simulink model "SF103A_MotorReferenceModel_v001B_MappedToEA4"  (R2013b)
settings: Solver=FixedStepDiscrete  StartTime=0.0  StopTime=10.0  RelTol=1e-3
InitFcn:
  | SF103A_MotorReferenceModel_v001X_Parameters;
undefined symbols (not defined in the file or in its folder): D_DTSCLMAX_ULS, D_DTSCLMIN_ULS, D_VECUMAX_VOLTS, D_VECUMIN_VOLTS, MtrCtrl_d_Ts_slow_s, MtrCtrl_e_KeNom_VpRadpS, MtrCtrl_e_RmNom_Ohm, MtrCtrl_k_deadtimeVScale_Uls, MtrCtrl_k_FeedbackControlDisable_Cnt, MtrCtrl_k_IdBoostGain_Uls, MtrCtrl_k_IdBoostVRThreshScl_Uls, MtrCtrl_k_IdqRefIminTol_Uls, MtrCtrl_k_IdqRefTrqTol_Uls, MtrCtrl_k_LdNom_Henry, MtrCtrl_k_LqNom_Henry, MtrCtrl_k_MtrCurrDaxMaxValScl_Per, MtrCtrl_k_MtrVoltDervFiltTimeConst_Sec, MtrCtrl_k_NoofPoles_Uls, MtrCtrl_k_VoltModeDynCompEnable_Cnt, MtrCtrl_t_IdBoostTrqCharSclY_Uls, MtrCtrl_t_IdBoostTrqCmdX_MtrNm, MtrCtrl_t_IdqRefDeltaPoints_Rad, MtrCtrl_t_Q13VltgSchedXTbl_MtrRadpS, MtrCtrl_t_Q13VltgSchedYTbl_Volt, MtrCtrl_t_Q24VltgSchedXTbl_MtrRadpS, MtrCtrl_t_Q24VltgSchedYTbl_Volt
undefined symbols (not defined in the file): MtrCtrl_k_MtrVelFiltFFKn_Hz
libraries: simulink x6
(part 2 of 2)

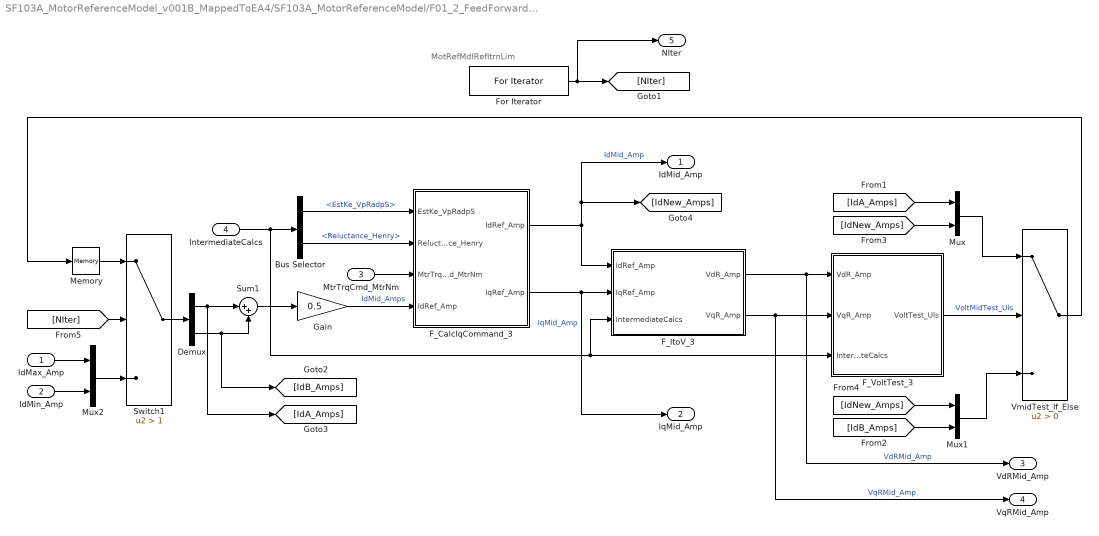
== system SF103A_MotorReferenceModel_v001B_MappedToEA4/SF103A_MotorReferenceModel/F01_2_FeedForward_Reference_Calc/F01_1_6_6_LocateRef/F01_1_6_6_1_ForIteratorSubsystem ==
  note: MotRefMdlRefItrnLim
  IdMax_Amp : Inport
  IdMin_Amp : Inport  Port=2
  MtrTrqCmd_MtrNm : Inport  Port=3
  IntermediateCalcs : Inport  Port=4
  Bus Selector : BusSelector  OutputSignals=EstKe_VpRadpS,Reluctance_Henry
  Demux : Demux  Outputs=2
  F_CalcIqCommand_3 : Subsystem
  F_ItoV_3 : Subsystem
  F_VoltTest_3 : Subsystem
  For Iterator : ForIterator  IterationLimit=MtrCtrl_k_IdqRefLocateRefNIter_Uls
  Gain : Gain  Gain=0.5
  Memory : Memory  InheritSampleTime=on
  Mux : Mux  Inputs=2
  Mux1 : Mux  Inputs=2
  Mux2 : Mux  Inputs=2
  Sum1 : Sum  Inputs=|++
  Switch1 : Switch  Criteria=u2 > Threshold  Threshold=1
  VmidTest_If_Else : Switch  Criteria=u2 > Threshold
  IdMid_Amp : Outport
  IqMid_Amp : Outport  Port=2
  VdRMid_Amp : Outport  Port=3
  VqRMid_Amp : Outport  Port=4
  NIter : Outport  Port=5
  wires:
  Sum1/1 -> Gain/1
  Demux/2 -> [IdB_Amps], Sum1/2
  Demux/1 -> [IdA_Amps], Sum1/1
  Switch1/1 -> Demux/1
  IdMax_Amp/1 -> Mux2/1
  Mux2/1 -> Switch1/3
  IdMin_Amp/1 -> Mux2/2
  [NIter] -> Switch1/2
  Memory/1 -> Switch1/1
  [IdB_Amps] -> Mux1/2
  [IdNew_Amps] -> Mux1/1
  [IdNew_Amps] -> Mux/2
  [IdA_Amps] -> Mux/1
  VmidTest_If_Else/1 -> Memory/1
  Mux1/1 -> VmidTest_If_Else/3
  Mux/1 -> VmidTest_If_Else/1
  For Iterator/1 -> NIter/1, [NIter]
  F_VoltTest_3/1(VoltTest_Uls) -> VmidTest_If_Else/2  "VoltMidTest_Uls"
  F_ItoV_3/2(VqR_Amp) -> F_VoltTest_3/2(VqR_Amp), VqRMid_Amp/1  "VqRMid_Amp"
  F_ItoV_3/1(VdR_Amp) -> F_VoltTest_3/1(VdR_Amp), VdRMid_Amp/1  "VdRMid_Amp"
  F_CalcIqCommand_3/2(IqRef_Amp) -> F_ItoV_3/2(IqRef_Amp), IqMid_Amp/1  "IqMid_Amp"
  F_CalcIqCommand_3/1(IdRef_Amp) -> F_ItoV_3/1(IdRef_Amp), IdMid_Amp/1, [IdNew_Amps]  "IdMid_Amp"
  MtrTrqCmd_MtrNm/1 -> F_CalcIqCommand_3/3(MtrTrqCmd_MtrNm)
  Bus Selector/2 -> F_CalcIqCommand_3/2(Reluctance_Henry)  "<Reluctance_Henry>"
  Bus Selector/1 -> F_CalcIqCommand_3/1(EstKe_VpRadpS)  "<EstKe_VpRadpS>"
  Gain/1 -> F_CalcIqCommand_3/4("IdRef_Amp ")  "IdMid_Amps"
  IntermediateCalcs/1 -> F_ItoV_3/3(IntermediateCalcs), F_VoltTest_3/3(IntermediateCalcs), Bus Selector/1

== system SF103A_MotorReferenceModel_v001B_MappedToEA4/SF103A_MotorReferenceModel/F01_2_FeedForward_Reference_Calc/F01_1_6_6_LocateRef/F_CalcIqCommand_1 ==
  EstKe_VpRadpS : Inport
  Reluctance_Henry : Inport  Port=2
  MtrTrqCmd_MtrNm : Inport  Port=3
  "IdRef_Amp " : Inport  Port=4
  Product : Product  RndMeth=Zero
  Product1 : Product  Inputs=*/  RndMeth=Zero
  Sum : Sum  Inputs=|++
  IdRef_Amp : Outport
  IqRef_Amp : Outport  Port=2
  wires:
  Product1/1 -> IqRef_Amp/1
  MtrTrqCmd_MtrNm/1 -> Product1/1
  Sum/1 -> Product1/2
  Product/1 -> Sum/2
  EstKe_VpRadpS/1 -> Sum/1
  "IdRef_Amp "/1 -> IdRef_Amp/1, Product/2
  Reluctance_Henry/1 -> Product/1

== system SF103A_MotorReferenceModel_v001B_MappedToEA4/SF103A_MotorReferenceModel/F01_2_FeedForward_Reference_Calc/F01_1_6_6_LocateRef/F_ItoV_1  ==
  IdRef_Amp : Inport
  IqRef_Amp : Inport  Port=2
  IntermediateCalcs : Inport  Port=3
  Bus Selector1 : BusSelector  OutputSignals=XqOvrR_Uls,XdOvrR_Uls,EgOvrR_Amp
  Product : Product  RndMeth=Zero
  Product1 : Product  RndMeth=Zero
  Sum : Sum  Inputs=|+-
  Sum1 : Sum  Inputs=+++
  VdR_Amp : Outport
  VqR_Amp : Outport  Port=2
  wires:
  IqRef_Amp/1 -> Product/1, Sum1/1
  IdRef_Amp/1 -> Sum/2, Product1/1
  IntermediateCalcs/1 -> Bus Selector1/1
  Bus Selector1/1 -> Product/2  "<XqOvrR_Uls>"
  Bus Selector1/2 -> Product1/2  "<XdOvrR_Uls>"
  Bus Selector1/3 -> Sum1/3  "<EgOvrR_Amp>"
  Product/1 -> Sum/1
  Sum/1 -> VdR_Amp/1
  Product1/1 -> Sum1/2
  Sum1/1 -> VqR_Amp/1

== system SF103A_MotorReferenceModel_v001B_MappedToEA4/SF103A_MotorReferenceModel/F01_2_FeedForward_Reference_Calc/F01_1_6_6_LocateRef/F_ItoV_2 ==
  IdRef_Amp : Inport
  IqRef_Amp : Inport  Port=2
  IntermediateCalcs : Inport  Port=3
  Bus Selector1 : BusSelector  OutputSignals=XqOvrR_Uls,XdOvrR_Uls,EgOvrR_Amp
  Product : Product  RndMeth=Zero
  Product1 : Product  RndMeth=Zero
  Sum : Sum  Inputs=|+-
  Sum1 : Sum  Inputs=+++
  VdR_Amp : Outport
  VqR_Amp : Outport  Port=2
  wires:
  Sum1/1 -> VqR_Amp/1
  Product1/1 -> Sum1/2
  Sum/1 -> VdR_Amp/1
  Product/1 -> Sum/1
  Bus Selector1/3 -> Sum1/3  "<EgOvrR_Amp>"
  Bus Selector1/2 -> Product1/2  "<XdOvrR_Uls>"
  Bus Selector1/1 -> Product/2  "<XqOvrR_Uls>"
  IntermediateCalcs/1 -> Bus Selector1/1
  IdRef_Amp/1 -> Product1/1, Sum/2
  IqRef_Amp/1 -> Sum1/1, Product/1

== system SF103A_MotorReferenceModel_v001B_MappedToEA4/SF103A_MotorReferenceModel/F01_2_FeedForward_Reference_Calc/F01_1_6_6_LocateRef/F_VoltTest_1 ==
  VdR_Amp : Inport
  VqR_Amp : Inport  Port=2
  IntermediateCalcs : Inport  Port=3
  Bus Selector1 : BusSelector  OutputSignals=VR2_AmpSq
  FALSE : Constant  Value=0
  Math Function : Math  Operator=square  SaturateOnIntegerOverflow=on
  Math Function1 : Math  Operator=square  SaturateOnIntegerOverflow=on
  Sum : Sum  Inputs=|++
  Sum1 : Sum  Inputs=-+|
  Switch : Switch
  TRUE : Constant
  VoltTest_Uls : Outport
  wires:
  IntermediateCalcs/1 -> Bus Selector1/1
  Bus Selector1/1 -> Sum1/1  "<VR2_AmpSq>"
  VdR_Amp/1 -> Math Function/1  "VdR_Amp"
  VqR_Amp/1 -> Math Function1/1  "VqR_Amp"
  Math Function/1 -> Sum/1
  Math Function1/1 -> Sum/2
  Sum/1 -> Sum1/2
  Sum1/1 -> Switch/2
  TRUE/1 -> Switch/1
  FALSE/1 -> Switch/3
  Switch/1 -> VoltTest_Uls/1

== system SF103A_MotorReferenceModel_v001B_MappedToEA4/SF103A_MotorReferenceModel/F01_2_FeedForward_Reference_Calc/F01_1_6_6_LocateRef/F_VoltTest_2 ==
  VdR_Amp : Inport
  VqR_Amp : Inport  Port=2
  IntermediateCalcs : Inport  Port=3
  Bus Selector1 : BusSelector  OutputSignals=VR2_AmpSq
  FALSE : Constant  Value=0
  Math Function : Math  Operator=square  SaturateOnIntegerOverflow=on
  Math Function1 : Math  Operator=square  SaturateOnIntegerOverflow=on
  Sum : Sum  Inputs=|++
  Sum1 : Sum  Inputs=-+|
  Switch : Switch
  TRUE : Constant
  VoltTest_Uls : Outport
  wires:
  Switch/1 -> VoltTest_Uls/1
  FALSE/1 -> Switch/3
  TRUE/1 -> Switch/1
  Sum1/1 -> Switch/2
  Sum/1 -> Sum1/2
  Math Function1/1 -> Sum/2
  Math Function/1 -> Sum/1
  VqR_Amp/1 -> Math Function1/1  "VqR_Amp"
  VdR_Amp/1 -> Math Function/1  "VdR_Amp"
  Bus Selector1/1 -> Sum1/1  "<VR2_AmpSq>"
  IntermediateCalcs/1 -> Bus Selector1/1

== system SF103A_MotorReferenceModel_v001B_MappedToEA4/SF103A_MotorReferenceModel/F01_2_FeedForward_Reference_Calc/F01_1_6_7_DAxisCurrentBoost/F_CalcIqCommand ==
  EstKe_VpRadpS : Inport
  Reluctance_Henry : Inport  Port=2
  MtrTrqCmd_MtrNm : Inport  Port=3
  "IdRef_Amp " : Inport  Port=4
  Product : Product  RndMeth=Zero
  Product1 : Product  Inputs=*/  RndMeth=Zero
  Sum : Sum  Inputs=|++
  IdRef_Amp : Outport
  IqRef_Amp : Outport  Port=2
  wires:
  Product1/1 -> IqRef_Amp/1
  MtrTrqCmd_MtrNm/1 -> Product1/1
  Sum/1 -> Product1/2
  Product/1 -> Sum/2
  EstKe_VpRadpS/1 -> Sum/1
  "IdRef_Amp "/1 -> IdRef_Amp/1, Product/2
  Reluctance_Henry/1 -> Product/1

== system SF103A_MotorReferenceModel_v001B_MappedToEA4/SF103A_MotorReferenceModel/F01_2_FeedForward_Reference_Calc/F01_1_6_7_DAxisCurrentBoost/F_ItoV  ==
  IdRef_Amp : Inport
  IqRef_Amp : Inport  Port=2
  IntermediateCalcs : Inport  Port=3
  Bus Selector1 : BusSelector  OutputSignals=XqOvrR_Uls,XdOvrR_Uls,EgOvrR_Amp
  Product : Product  RndMeth=Zero
  Product1 : Product  RndMeth=Zero
  Sum : Sum  Inputs=|+-
  Sum1 : Sum  Inputs=+++
  VdR_Amp : Outport
  VqR_Amp : Outport  Port=2
  wires:
  IqRef_Amp/1 -> Product/1, Sum1/1
  IdRef_Amp/1 -> Sum/2, Product1/1
  IntermediateCalcs/1 -> Bus Selector1/1
  Bus Selector1/1 -> Product/2  "<XqOvrR_Uls>"
  Bus Selector1/2 -> Product1/2  "<XdOvrR_Uls>"
  Bus Selector1/3 -> Sum1/3  "<EgOvrR_Amp>"
  Product/1 -> Sum/1
  Sum/1 -> VdR_Amp/1
  Product1/1 -> Sum1/2
  Sum1/1 -> VqR_Amp/1

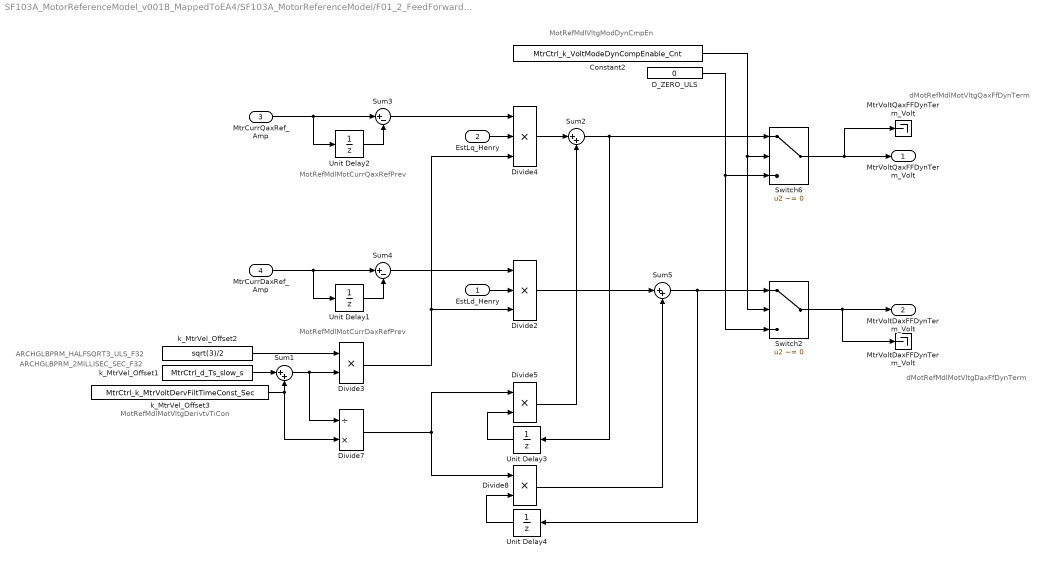
== system SF103A_MotorReferenceModel_v001B_MappedToEA4/SF103A_MotorReferenceModel/F01_2_FeedForward_Reference_Calc/F01_1_6_8_FeedforwardVoltage/F01_1_6_8_1_DynamicTermCalc ==
  note: MotRefMdlMotCurrQaxRefPrev
  note: MotRefMdlVltgModDynCmpEn
  note: MotRefMdlMotVltgDerivtvTiCon
  note: dMotRefMdlMotVltgQaxFfDynTerm
  note: dMotRefMdlMotVltgDaxFfDynTerm
  note: MotRefMdlMotCurrDaxRefPrev
  note: ARCHGLBPRM_HALFSQRT3_ULS_F32
  note: ARCHGLBPRM_2MILLISEC_SEC_F32
  EstLd_Henry : Inport
  EstLq_Henry : Inport  Port=2
  MtrCurrQaxRef_Amp : Inport  Port=3
  MtrCurrDaxRef_Amp : Inport  Port=4
  Constant2 : Constant  Value=MtrCtrl_k_VoltModeDynCompEnable_Cnt
  D_ZERO_ULS : Constant  Value=0
  Divide2 : Product  Inputs=3
  Divide3 : Product
  Divide4 : Product  Inputs=3
  Divide5 : Product
  Divide7 : Product  Inputs=/*
  Divide8 : Product
  "MtrVoltDaxFFDynTerm_Volt " : Terminator
  "MtrVoltQaxFFDynTerm_Volt " : Terminator
  Sum1 : Sum  Inputs=|++
  Sum2 : Sum  Inputs=|++
  Sum3 : Sum  Inputs=|+-
  Sum4 : Sum  Inputs=|+-
  Sum5 : Sum  Inputs=|++
  Switch2 : Switch  Criteria=u2 ~= 0
  Switch6 : Switch  Criteria=u2 ~= 0
  Unit Delay{1..4} (4 alike) : UnitDelay  SampleTime=-1
  k_MtrVel_Offset1 : Constant  Value=MtrCtrl_d_Ts_slow_s  SampleTime=MtrCtrl_d_Ts_slow_s
  k_MtrVel_Offset2 : Constant  Value=sqrt(3)/2  SampleTime=MtrCtrl_d_Ts_slow_s
  k_MtrVel_Offset3 : Constant  Value=MtrCtrl_k_MtrVoltDervFiltTimeConst_Sec  SampleTime=MtrCtrl_d_Ts_slow_s
  MtrVoltQaxFFDynTerm_Volt : Outport
  MtrVoltDaxFFDynTerm_Volt : Outport  Port=2
  wires:
  Sum2/1 -> Unit Delay3/1, Switch6/1
  EstLd_Henry/1 -> Divide2/2
  k_MtrVel_Offset2/1 -> Divide3/1
  k_MtrVel_Offset1/1 -> Sum1/1
  Sum1/1 -> Divide7/1, Divide3/2
  k_MtrVel_Offset3/1 -> Divide7/2, Sum1/2
  EstLq_Henry/1 -> Divide4/2
  Divide3/1 -> Divide4/3, Divide2/3
  Divide4/1 -> Sum2/1
  MtrCurrQaxRef_Amp/1 -> Unit Delay2/1, Sum3/1
  Unit Delay2/1 -> Sum3/2
  Sum3/1 -> Divide4/1
  MtrCurrDaxRef_Amp/1 -> Sum4/1, Unit Delay1/1
  Unit Delay1/1 -> Sum4/2
  Sum4/1 -> Divide2/1
  Divide7/1 -> Divide5/1, Divide8/1
  Divide5/1 -> Sum2/2
  Unit Delay3/1 -> Divide5/2
  Divide2/1 -> Sum5/1
  Unit Delay4/1 -> Divide8/2
  Divide8/1 -> Sum5/2
  Sum5/1 -> Unit Delay4/1, Switch2/1
  Constant2/1 -> Switch2/2, Switch6/2
  D_ZERO_ULS/1 -> Switch6/3, Switch2/3
  Switch6/1 -> "MtrVoltQaxFFDynTerm_Volt "/1, MtrVoltQaxFFDynTerm_Volt/1
  Switch2/1 -> "MtrVoltDaxFFDynTerm_Volt "/1, MtrVoltDaxFFDynTerm_Volt/1

== system SF103A_MotorReferenceModel_v001B_MappedToEA4/SF103A_MotorReferenceModel/F01_2_FeedForward_Reference_Calc/F01_1_6_8_FeedforwardVoltage/F01_1_6_8_2_FeedforwardSelection ==
  note: MotRefMdlFbCtrlDi
  note: dMotRefMdlMotVltgQaxFfDyn
  note: dMotRefMdlMotVltgDaxFfDyn
  MtrVoltDaxFFStatic_Volt : Inport
  MtrVoltQaxFFStatic_Volt : Inport  Port=2
  FailOperActive_Cnt : Inport  Port=3
  MtrVoltQaxFFDynTerm_Volt : Inport  Port=4
  MtrVoltDaxFFDynTerm_Volt : Inport  Port=5
  IntermediateCalcs : Inport  Port=6
  Bus Selector : BusSelector  OutputSignals=EgOvrR_Amp,EstR_Ohm
  D_ZERO_ULS : Constant  Value=0  SampleTime=MtrCtrl_d_Ts_slow_s
  Logical Operator : Logic  Operator=OR  AllPortsSameDT=off  OutDataTypeStr=boolean
  MtrVoltDaxFFDynamic_Volt : Terminator
  "MtrVoltDaxFF_Volt " : Terminator
  MtrVoltQaxFFDynamic_Volt : Terminator
  "MtrVoltQaxFF_Volt " : Terminator
  Product : Product  RndMeth=Zero
  Sum1 : Sum  Inputs=|++
  Sum5 : Sum  Inputs=|++
  Switch1 : Switch  Criteria=u2 ~= 0  SampleTime=MtrCtrl_d_Ts_slow_s
  Switch4 : Switch  Criteria=u2 ~= 0  SampleTime=MtrCtrl_d_Ts_slow_s
  k_MtrVel_Offset9 : Constant  Value=MtrCtrl_k_FeedbackControlDisable_Cnt  SampleTime=MtrCtrl_d_Ts_slow_s
  MtrVoltDaxFF_Volt : Outport
  MtrVoltQaxFF_Volt : Outport  Port=2
  wires:
  Sum5/1 -> Switch1/1, MtrVoltDaxFFDynamic_Volt/1
  Sum1/1 -> MtrVoltQaxFFDynamic_Volt/1, Switch4/1
  Logical Operator/1 -> Switch1/2, Switch4/2
  Switch1/1 -> "MtrVoltDaxFF_Volt "/1, MtrVoltDaxFF_Volt/1
  Switch4/1 -> "MtrVoltQaxFF_Volt "/1, MtrVoltQaxFF_Volt/1
  Product/1 -> Switch4/3
  Bus Selector/2 -> Product/2  "<EstR_Ohm>"
  Bus Selector/1 -> Product/1  "<EgOvrR_Amp>"
  IntermediateCalcs/1 -> Bus Selector/1
  D_ZERO_ULS/1 -> Switch1/3
  k_MtrVel_Offset9/1 -> Logical Operator/1
  FailOperActive_Cnt/1 -> Logical Operator/2
  MtrVoltDaxFFStatic_Volt/1 -> Sum5/1
  MtrVoltDaxFFDynTerm_Volt/1 -> Sum5/2
  MtrVoltQaxFFDynTerm_Volt/1 -> Sum1/2
  MtrVoltQaxFFStatic_Volt/1 -> Sum1/1

== system SF103A_MotorReferenceModel_v001B_MappedToEA4/SF103A_MotorReferenceModel/F01_2_FeedForward_Reference_Calc/F01_1_6_3_LocateTorqueExtremes/F01_1_6_3_3_ChooseDeltaBrackets/F_CalculateTorque ==
  Current : Inport
  IntermediateCalcs : Inport  Port=2
  Bus Selector : BusSelector  OutputSignals=EstKe_VpRadpS,Reluctance_Henry
  Bus Selector1 : BusSelector  OutputSignals=IdRef_Amp,IqRef_Amp
  Product : Product  RndMeth=Zero
  Product1 : Product  RndMeth=Zero
  Sum : Sum  Inputs=++|
  Torque_MtrNm : Outport
  wires:
  Product1/1 -> Torque_MtrNm/1
  Sum/1 -> Product1/1
  Bus Selector1/2 -> Product1/2  "<IqRef_Amp>"
  Bus Selector1/1 -> Product/2  "<IdRef_Amp>"
  Product/1 -> Sum/2
  Current/1 -> Bus Selector1/1
  Bus Selector/2 -> Product/1  "<Reluctance_Henry>"
  Bus Selector/1 -> Sum/1  "<EstKe_VpRadpS>"
  IntermediateCalcs/1 -> Bus Selector/1

== system SF103A_MotorReferenceModel_v001B_MappedToEA4/SF103A_MotorReferenceModel/F01_2_FeedForward_Reference_Calc/F01_1_6_3_LocateTorqueExtremes/F01_1_6_3_3_ChooseDeltaBrackets/F_VSinCosToIdIq ==
  SinDelta : Inport
  CosDelta : Inport  Port=2
  IntermediateCalcs : Inport  Port=3
  Bus Creator : BusCreator  Inputs=2
  Bus Selector2 : BusSelector  OutputSignals=XdOvrR_Uls,VOvrROvrZ_Amp,EgOvrROvrZ_Amp,XqOvrR_Uls,VOvrR_Amp
  Product{,1..3} (4 alike) : Product  RndMeth=Zero
  Sum : Sum  Inputs=|++
  Sum1 : Sum  Inputs=|+-
  Sum2 : Sum  Inputs=|+-
  IdIq_Amp : Outport
  wires:
  Bus Creator/1 -> IdIq_Amp/1
  Sum2/1 -> Bus Creator/2  "IdRef_Amp"
  Product3/1 -> Sum2/2
  Product2/1 -> Sum2/1
  Sum1/1 -> Bus Creator/1, Product2/1  "IqRef_Amp"
  Product1/1 -> Sum1/1
  Sum/1 -> Product1/1
  Product/1 -> Sum/1
  CosDelta/1 -> Sum/2
  SinDelta/1 -> Product3/2, Product/1
  Bus Selector2/5 -> Product3/1  "<VOvrR_Amp>"
  Bus Selector2/4 -> Product2/2  "<XqOvrR_Uls>"
  Bus Selector2/3 -> Sum1/2  "<EgOvrROvrZ_Amp>"
  Bus Selector2/1 -> Product/2  "<XdOvrR_Uls>"
  Bus Selector2/2 -> Product1/2  "<VOvrROvrZ_Amp>"
  IntermediateCalcs/1 -> Bus Selector2/1

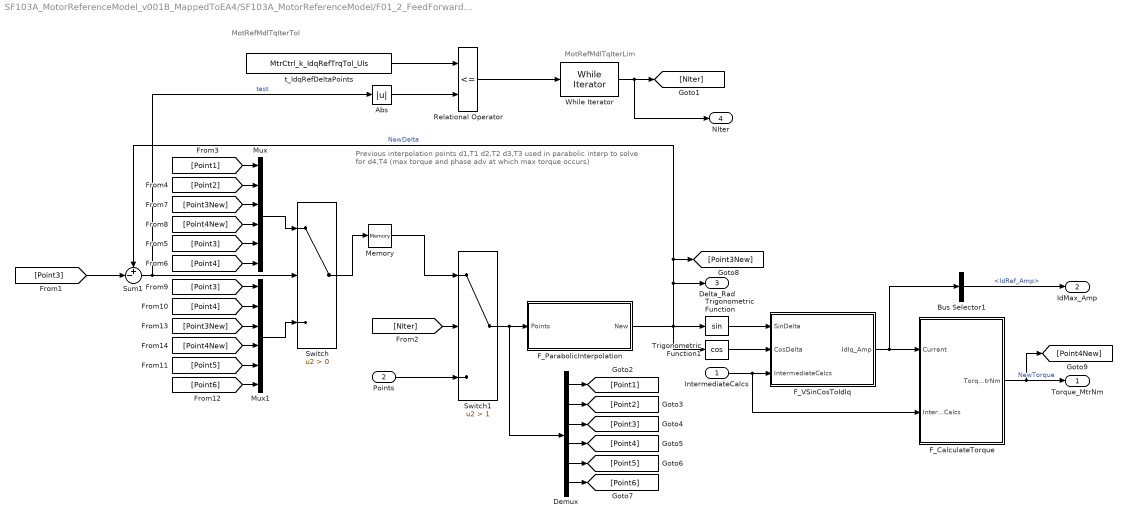
== system SF103A_MotorReferenceModel_v001B_MappedToEA4/SF103A_MotorReferenceModel/F01_2_FeedForward_Reference_Calc/F01_1_6_3_LocateTorqueExtremes/F01_1_6_3_5_InterpolatePeakTorque/F01_1_6_3_5_1_WhileIteratorSubsystem ==
  note: MotRefMdlTqIterLim
  note: Previous interpolation points
      | d1,T1
      | d2,T2
      | d3,T3
      | used in parabolic interp to solve for
      | d4,T4 (max torque and phase adv at which max torque occurs)
  note: MotRefMdlTqIterTol
  IntermediateCalcs : Inport
  Points : Inport  Port=2
  Abs : Abs
  Bus Selector1 : BusSelector  OutputSignals=IdRef_Amp
  Demux : Demux  Outputs=6
  F_CalculateTorque : Subsystem
  F_ParabolicInterpolation : Subsystem
  F_VSinCosToIdIq : Subsystem
  Memory : Memory  InheritSampleTime=on
  Mux : Mux  Inputs=6
  Mux1 : Mux  Inputs=6
  Relational Operator : RelationalOperator  Operator=<=  OutDataTypeStr=boolean
  Sum1 : Sum  Inputs=+-|
  Switch : Switch  Criteria=u2 > Threshold
  Switch1 : Switch  Criteria=u2 > Threshold  Threshold=1
  Trigonometric Function : Trigonometry
  Trigonometric Function1 : Trigonometry  Operator=cos
  While Iterator : WhileIterator  MaxIters=MtrCtrl_k_IdqRefTrqNIter_Uls  WhileBlockType=do-while  ShowIterationPort=on
  t_IdqRefDeltaPoints : Constant  Value=MtrCtrl_k_IdqRefTrqTol_Uls
  Torque_MtrNm : Outport
  IdMax_Amp : Outport  Port=2
  Delta_Rad : Outport  Port=3
  NIter : Outport  Port=4
  wires:
  t_IdqRefDeltaPoints/1 -> Relational Operator/1
  Mux1/1 -> Switch/3
  [Point4New] -> Mux1/4
  [Point3New] -> Mux1/3
  [Point6] -> Mux1/6
  [Point5] -> Mux1/5
  [Point3] -> Mux1/1
  [Point4] -> Mux1/2
  [Point4New] -> Mux/4
  [Point3New] -> Mux/3
  [Point4] -> Mux/6
  [Point3] -> Mux/5
  [Point1] -> Mux/1
  [Point2] -> Mux/2
  [Point3] -> Sum1/2
  Demux/6 -> [Point6]
  Demux/5 -> [Point5]
  Demux/4 -> [Point4]
  Demux/3 -> [Point3]
  Demux/2 -> [Point2]
  Demux/1 -> [Point1]
  Memory/1 -> Switch1/1
  Bus Selector1/1 -> IdMax_Amp/1  "<IdRef_Amp>"
  Points/1 -> Switch1/3
  [NIter] -> Switch1/2
  Switch1/1 -> F_ParabolicInterpolation/1(Points), Demux/1
  While Iterator/1 -> NIter/1, [NIter]
  Switch/1 -> Memory/1
  Mux/1 -> Switch/1
  F_CalculateTorque/1(Torque_MtrNm) -> [Point4New], Torque_MtrNm/1  "NewTorque"
  Abs/1 -> Relational Operator/2
  Sum1/1 -> Abs/1, Switch/2  "test"
  F_VSinCosToIdIq/1(IdIq_Amp) -> Bus Selector1/1, F_CalculateTorque/1(Current)
  IntermediateCalcs/1 -> F_CalculateTorque/2(IntermediateCalcs), F_VSinCosToIdIq/3(IntermediateCalcs)
  Trigonometric Function1/1 -> F_VSinCosToIdIq/2(CosDelta)
  Trigonometric Function/1 -> F_VSinCosToIdIq/1(SinDelta)
  F_ParabolicInterpolation/1(New) -> Trigonometric Function1/1, Sum1/1, [Point3New], Delta_Rad/1, Trigonometric Function/1  "NewDelta"
  Relational Operator/1 -> While Iterator/1

== system SF103A_MotorReferenceModel_v001B_MappedToEA4/SF103A_MotorReferenceModel/F01_2_FeedForward_Reference_Calc/F01_1_6_5_LocateMinIm/F01_1_6_5_1_WhileIteratorSubsystem/F_CalcIqCommand_3 ==
  EstKe_VpRadpS : Inport
  Reluctance_Henry : Inport  Port=2
  MtrTrqCmd_MtrNm : Inport  Port=3
  "IdRef_Amp " : Inport  Port=4
  Product : Product  RndMeth=Zero
  Product1 : Product  Inputs=*/  RndMeth=Zero
  Sum : Sum  Inputs=|++
  IdRef_Amp : Outport
  IqRef_Amp : Outport  Port=2
  wires:
  Reluctance_Henry/1 -> Product/1
  "IdRef_Amp "/1 -> Product/2, IdRef_Amp/1
  EstKe_VpRadpS/1 -> Sum/1
  Product/1 -> Sum/2
  Sum/1 -> Product1/2
  MtrTrqCmd_MtrNm/1 -> Product1/1
  Product1/1 -> IqRef_Amp/1

== system SF103A_MotorReferenceModel_v001B_MappedToEA4/SF103A_MotorReferenceModel/F01_2_FeedForward_Reference_Calc/F01_1_6_5_LocateMinIm/F01_1_6_5_1_WhileIteratorSubsystem/F_ImVSIdq_3 ==
  IdRef_Amp : Inport
  IqRef_Amp : Inport  Port=2
  Math Function : Math  Operator=square  SaturateOnIntegerOverflow=on
  Math Function1 : Math  Operator=square  SaturateOnIntegerOverflow=on
  Sum : Sum  Inputs=|++
  ImRefSq_AmpSq : Outport
  wires:
  IqRef_Amp/1 -> Math Function/1
  IdRef_Amp/1 -> Math Function1/1
  Math Function/1 -> Sum/1
  Math Function1/1 -> Sum/2
  Sum/1 -> ImRefSq_AmpSq/1

== system SF103A_MotorReferenceModel_v001B_MappedToEA4/SF103A_MotorReferenceModel/F01_2_FeedForward_Reference_Calc/F01_1_6_5_LocateMinIm/F01_1_6_5_1_WhileIteratorSubsystem/F_ParabolicInterpolation ==
  note: ARCHGLBPRM_FLOATZEROTHD_ULS_F32
  note: This function checks for
      | divide-by-zero condition
  Points : Inport
  Constant : Constant  Value=eps
  Demux : Demux  Outputs=6
  Gain : Gain  Gain=0.5
  Math Function : Math  Operator=square  SaturateOnIntegerOverflow=on
  Math Function1 : Math  Operator=square  SaturateOnIntegerOverflow=on
  Product{,1..3} (4 alike) : Product  RndMeth=Zero
  Product4 : Product  Inputs=*/  RndMeth=Zero
  Sum{,1..3,5} (5 alike) : Sum  Inputs=|+-
  Sum4 : Sum  Inputs=|++
  Sum6 : Sum  Inputs=|++
  Switch : Switch  Criteria=u2 ~= 0
  New : Outport
  wires:
  Switch/1 -> Product4/2
  Product4/1 -> Gain/1
  Constant/1 -> Switch/3
  Sum5/1 -> Switch/2, Switch/1  "den"
  Points/1 -> Demux/1
  Sum6/1 -> New/1
  Demux/2 -> Sum/1  "Point2:Torque"
  Demux/6 -> Sum1/2  "Point6:Torque"
  Demux/5 -> Sum3/2  "Point5:Delta"
  Demux/4 -> Sum/2, Sum1/1  "Point4:Torque"
  Demux/3 -> Sum3/1, Sum2/2, Sum6/2  "Point3:Delta"
  Demux/1 -> Sum2/1  "Point1:Delta"
  Gain/1 -> Sum6/1
  Product3/1 -> Sum5/2  "den2"
  Product2/1 -> Sum5/1  "den1"
  Sum4/1 -> Product4/1  "num"
  Product1/1 -> Sum4/2  "num2"
  Math Function1/1 -> Product1/2
  Product/1 -> Sum4/1  "num1"
  Math Function/1 -> Product/1
  Sum3/1 -> Product3/2, Math Function1/1  "x2"
  Sum2/1 -> Product2/2, Math Function/1  "x1"
  Sum1/1 -> Product2/1, Product/2  "f2"
  Sum/1 -> Product3/1, Product1/1  "f1"

== system SF103A_MotorReferenceModel_v001B_MappedToEA4/SF103A_MotorReferenceModel/F01_2_FeedForward_Reference_Calc/F01_1_6_6_LocateRef/F01_1_6_6_1_ForIteratorSubsystem/F_CalcIqCommand_3 ==
  EstKe_VpRadpS : Inport
  Reluctance_Henry : Inport  Port=2
  MtrTrqCmd_MtrNm : Inport  Port=3
  "IdRef_Amp " : Inport  Port=4
  Product : Product  RndMeth=Zero
  Product1 : Product  Inputs=*/  RndMeth=Zero
  Sum : Sum  Inputs=|++
  IdRef_Amp : Outport
  IqRef_Amp : Outport  Port=2
  wires:
  Reluctance_Henry/1 -> Product/1
  "IdRef_Amp "/1 -> Product/2, IdRef_Amp/1
  EstKe_VpRadpS/1 -> Sum/1
  Product/1 -> Sum/2
  Sum/1 -> Product1/2
  MtrTrqCmd_MtrNm/1 -> Product1/1
  Product1/1 -> IqRef_Amp/1

== system SF103A_MotorReferenceModel_v001B_MappedToEA4/SF103A_MotorReferenceModel/F01_2_FeedForward_Reference_Calc/F01_1_6_6_LocateRef/F01_1_6_6_1_ForIteratorSubsystem/F_ItoV_3 ==
  IdRef_Amp : Inport
  IqRef_Amp : Inport  Port=2
  IntermediateCalcs : Inport  Port=3
  Bus Selector1 : BusSelector  OutputSignals=XqOvrR_Uls,XdOvrR_Uls,EgOvrR_Amp
  Product : Product  RndMeth=Zero
  Product1 : Product  RndMeth=Zero
  Sum : Sum  Inputs=|+-
  Sum1 : Sum  Inputs=+++
  VdR_Amp : Outport
  VqR_Amp : Outport  Port=2
  wires:
  IqRef_Amp/1 -> Product/1, Sum1/1
  IdRef_Amp/1 -> Sum/2, Product1/1
  IntermediateCalcs/1 -> Bus Selector1/1
  Bus Selector1/1 -> Product/2  "<XqOvrR_Uls>"
  Bus Selector1/2 -> Product1/2  "<XdOvrR_Uls>"
  Bus Selector1/3 -> Sum1/3  "<EgOvrR_Amp>"
  Product/1 -> Sum/1
  Sum/1 -> VdR_Amp/1
  Product1/1 -> Sum1/2
  Sum1/1 -> VqR_Amp/1

== system SF103A_MotorReferenceModel_v001B_MappedToEA4/SF103A_MotorReferenceModel/F01_2_FeedForward_Reference_Calc/F01_1_6_6_LocateRef/F01_1_6_6_1_ForIteratorSubsystem/F_VoltTest_3 ==
  VdR_Amp : Inport
  VqR_Amp : Inport  Port=2
  IntermediateCalcs : Inport  Port=3
  Bus Selector1 : BusSelector  OutputSignals=VR2_AmpSq
  FALSE : Constant  Value=0
  Math Function : Math  Operator=square  SaturateOnIntegerOverflow=on
  Math Function1 : Math  Operator=square  SaturateOnIntegerOverflow=on
  Sum : Sum  Inputs=|++
  Sum1 : Sum  Inputs=-+|
  Switch : Switch
  TRUE : Constant
  VoltTest_Uls : Outport
  wires:
  IntermediateCalcs/1 -> Bus Selector1/1
  Bus Selector1/1 -> Sum1/1  "<VR2_AmpSq>"
  VdR_Amp/1 -> Math Function/1  "VdR_Amp"
  VqR_Amp/1 -> Math Function1/1  "VqR_Amp"
  Math Function/1 -> Sum/1
  Math Function1/1 -> Sum/2
  Sum/1 -> Sum1/2
  Sum1/1 -> Switch/2
  TRUE/1 -> Switch/1
  FALSE/1 -> Switch/3
  Switch/1 -> VoltTest_Uls/1

== system SF103A_MotorReferenceModel_v001B_MappedToEA4/SF103A_MotorReferenceModel/F01_2_FeedForward_Reference_Calc/F01_1_6_3_LocateTorqueExtremes/F01_1_6_3_5_InterpolatePeakTorque/F01_1_6_3_5_1_WhileIteratorSubsystem/F_CalculateTorque ==
  Current : Inport
  IntermediateCalcs : Inport  Port=2
  Bus Selector : BusSelector  OutputSignals=EstKe_VpRadpS,Reluctance_Henry
  Bus Selector1 : BusSelector  OutputSignals=IdRef_Amp,IqRef_Amp
  Product : Product  RndMeth=Zero
  Product1 : Product  RndMeth=Zero
  Sum : Sum  Inputs=++|
  Torque_MtrNm : Outport
  wires:
  Product1/1 -> Torque_MtrNm/1
  Sum/1 -> Product1/1
  Bus Selector1/2 -> Product1/2  "<IqRef_Amp>"
  Bus Selector1/1 -> Product/2  "<IdRef_Amp>"
  Product/1 -> Sum/2
  Current/1 -> Bus Selector1/1
  Bus Selector/2 -> Product/1  "<Reluctance_Henry>"
  Bus Selector/1 -> Sum/1  "<EstKe_VpRadpS>"
  IntermediateCalcs/1 -> Bus Selector/1

== system SF103A_MotorReferenceModel_v001B_MappedToEA4/SF103A_MotorReferenceModel/F01_2_FeedForward_Reference_Calc/F01_1_6_3_LocateTorqueExtremes/F01_1_6_3_5_InterpolatePeakTorque/F01_1_6_3_5_1_WhileIteratorSubsystem/F_ParabolicInterpolation ==
  note: What is "eps"?
      | It's not in Prerit parameter file.
  note: This function checks for
      | divide-by-zero condition
  Points : Inport
  Constant : Constant  Value=eps
  Demux : Demux  Outputs=6
  Gain : Gain  Gain=0.5
  Math Function : Math  Operator=square  SaturateOnIntegerOverflow=on
  Math Function1 : Math  Operator=square  SaturateOnIntegerOverflow=on
  Product{,1..3} (4 alike) : Product  RndMeth=Zero
  Product4 : Product  Inputs=*/  RndMeth=Zero
  Sum{,1..3,5} (5 alike) : Sum  Inputs=|+-
  Sum4 : Sum  Inputs=|++
  Sum6 : Sum  Inputs=|++
  Switch : Switch  Criteria=u2 ~= 0
  New : Outport
  wires:
  Switch/1 -> Product4/2
  Product4/1 -> Gain/1
  Constant/1 -> Switch/3
  Sum5/1 -> Switch/2, Switch/1  "den"
  Points/1 -> Demux/1
  Sum6/1 -> New/1
  Demux/2 -> Sum/1  "Point2:Torque"
  Demux/6 -> Sum1/2  "Point6:Torque"
  Demux/5 -> Sum3/2  "Point5:Delta"
  Demux/4 -> Sum/2, Sum1/1  "Point4:Torque"
  Demux/3 -> Sum3/1, Sum2/2, Sum6/2  "Point3:Delta"
  Demux/1 -> Sum2/1  "Point1:Delta"
  Gain/1 -> Sum6/1
  Product3/1 -> Sum5/2  "den2"
  Product2/1 -> Sum5/1  "den1"
  Sum4/1 -> Product4/1  "num"
  Product1/1 -> Sum4/2  "num2"
  Math Function1/1 -> Product1/2
  Product/1 -> Sum4/1  "num1"
  Math Function/1 -> Product/1
  Sum3/1 -> Product3/2, Math Function1/1  "x2"
  Sum2/1 -> Product2/2, Math Function/1  "x1"
  Sum1/1 -> Product2/1, Product/2  "f2"
  Sum/1 -> Product3/1, Product1/1  "f1"

== system SF103A_MotorReferenceModel_v001B_MappedToEA4/SF103A_MotorReferenceModel/F01_2_FeedForward_Reference_Calc/F01_1_6_3_LocateTorqueExtremes/F01_1_6_3_5_InterpolatePeakTorque/F01_1_6_3_5_1_WhileIteratorSubsystem/F_VSinCosToIdIq ==
  SinDelta : Inport
  CosDelta : Inport  Port=2
  IntermediateCalcs : Inport  Port=3
  Bus Creator : BusCreator  Inputs=2
  Bus Selector2 : BusSelector  OutputSignals=XdOvrR_Uls,VOvrROvrZ_Amp,EgOvrROvrZ_Amp,XqOvrR_Uls,VOvrR_Amp
  Product{,1..3} (4 alike) : Product  RndMeth=Zero
  Sum : Sum  Inputs=|++
  Sum1 : Sum  Inputs=|+-
  Sum2 : Sum  Inputs=|+-
  IdIq_Amp : Outport
  wires:
  Bus Creator/1 -> IdIq_Amp/1
  Sum2/1 -> Bus Creator/2  "IdRef_Amp"
  Product3/1 -> Sum2/2
  Product2/1 -> Sum2/1
  Sum1/1 -> Bus Creator/1, Product2/1  "IqRef_Amp"
  Product1/1 -> Sum1/1
  Sum/1 -> Product1/1
  Product/1 -> Sum/1
  CosDelta/1 -> Sum/2
  SinDelta/1 -> Product3/2, Product/1
  Bus Selector2/5 -> Product3/1  "<VOvrR_Amp>"
  Bus Selector2/4 -> Product2/2  "<XqOvrR_Uls>"
  Bus Selector2/3 -> Sum1/2  "<EgOvrROvrZ_Amp>"
  Bus Selector2/1 -> Product/2  "<XdOvrR_Uls>"
  Bus Selector2/2 -> Product1/2  "<VOvrROvrZ_Amp>"
  IntermediateCalcs/1 -> Bus Selector2/1
